simulink model "Load_Torque"  (R2025b)
settings: Solver=FixedStepAuto  StartTime=0.0  StopTime=10.0  FixedStep=0.001  RelTol=1e-3
undefined symbols (not defined in the file): nu_gen
settings Model: Creator=andre  LastModifiedBy=khanh

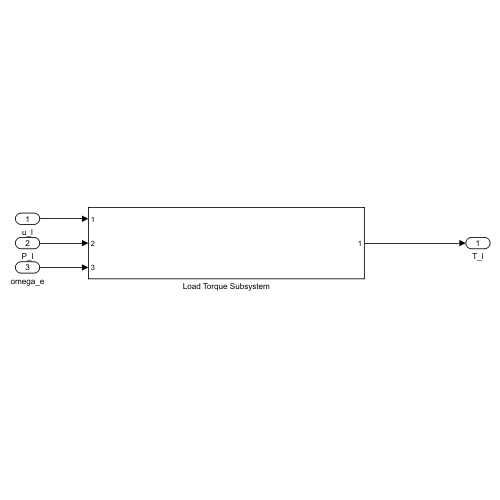
[thumbnail: Simulink's stored preview of the top-level diagram]
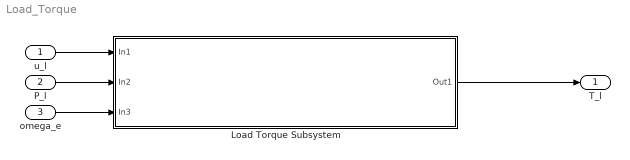
== system Load_Torque ==
  u_l : Inport
  P_l : Inport  Port=2
  omega_e : Inport  Port=3
  Load Torque Subsystem : Subsystem
  T_l : Outport
  wires:
  u_l/1 -> Load Torque Subsystem/1(In1)
  P_l/1 -> Load Torque Subsystem/2(In2)
  omega_e/1 -> Load Torque Subsystem/3(In3)
  Load Torque Subsystem/1(Out1) -> T_l/1

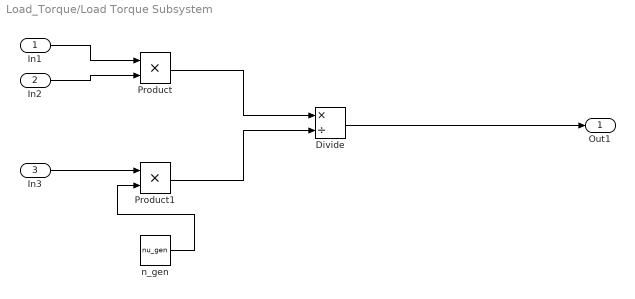
== system Load_Torque/Load Torque Subsystem ==
  In1 : Inport
  In2 : Inport  Port=2
  In3 : Inport  Port=3
  Divide : Product  Inputs=*/
  Product : Product
  Product1 : Product
  n_gen : Constant  Value=nu_gen
  Out1 : Outport
  wires:
  In2/1 -> Product/2
  In1/1 -> Product/1
  In3/1 -> Product1/1
  n_gen/1 -> Product1/2
  Divide/1 -> Out1/1
  Product/1 -> Divide/1
  Product1/1 -> Divide/2
